simulink model "CognitiveOperatorBackup"  (R2017a)
settings: Solver=VariableStepAuto  StartTime=0.0  StopTime=81  RelTol=1e-3
libraries: simulink x1
settings Model: PauseTimes=1  Creator=Igor Khimchenko  LastModifiedBy=Igor Khimchenko

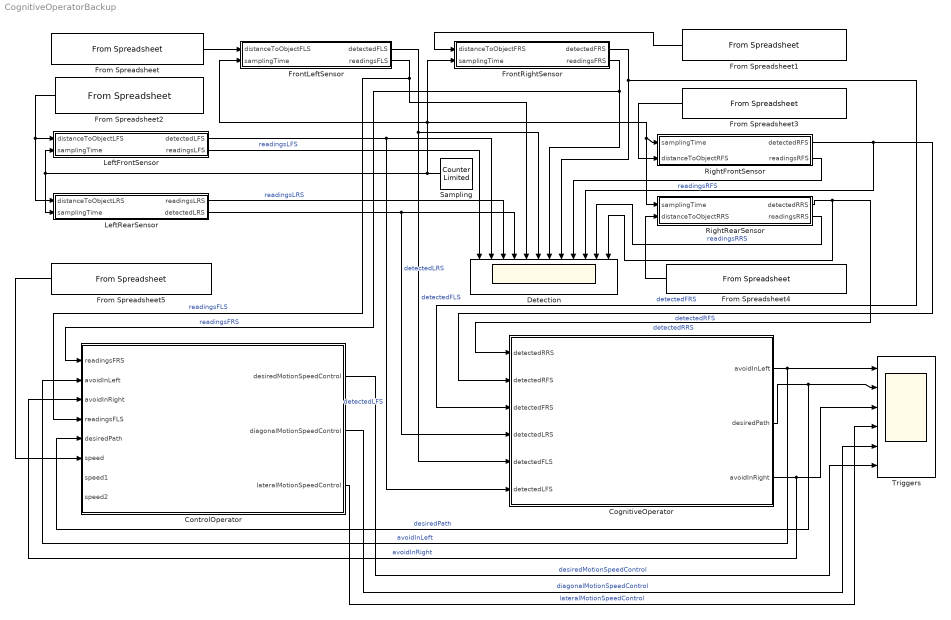
== system CognitiveOperatorBackup ==
  CognitiveOperator : Stateflow chart  TreatAsAtomicUnit=on
  ControlOperator : Stateflow chart  TreatAsAtomicUnit=on
  Detection : Scope  NumInputPorts=12
  From Spreadsheet : FromSpreadsheet  FileName=SensorReadings.xlsx  SheetName=Front left
  From Spreadsheet1 : FromSpreadsheet  FileName=SensorReadings.xlsx  SheetName=Front right
  From Spreadsheet2 : FromSpreadsheet  FileName=SensorReadings.xlsx  SheetName=Left
  From Spreadsheet3 : FromSpreadsheet  FileName=SensorReadings.xlsx  SheetName=Right front
  From Spreadsheet4 : FromSpreadsheet  FileName=SensorReadings.xlsx  SheetName=Right rear
  From Spreadsheet5 : FromSpreadsheet  FileName=SensorReadings.xlsx  SheetName=Speed
  FrontLeftSensor : Stateflow chart  TreatAsAtomicUnit=on
  FrontRightSensor : Stateflow chart  TreatAsAtomicUnit=on
  LeftFrontSensor : Stateflow chart  TreatAsAtomicUnit=on
  LeftRearSensor : Stateflow chart  TreatAsAtomicUnit=on
  RightFrontSensor : Stateflow chart  TreatAsAtomicUnit=on
  RightRearSensor : Stateflow chart  TreatAsAtomicUnit=on
  Sampling : simulink/Sources/Counter Limited  uplimit=50  tsamp=0.001
  Triggers : Scope  NumInputPorts=6
  wires:
  From Spreadsheet2/1 -> LeftRearSensor/1(distanceToObjectLRS), LeftFrontSensor/1(distanceToObjectLFS)
  Sampling/1 -> LeftRearSensor/2(samplingTime), LeftFrontSensor/2(samplingTime), FrontRightSensor/2(samplingTime), RightRearSensor/1(samplingTime), RightFrontSensor/1(samplingTime), FrontLeftSensor/2(samplingTime)
  LeftFrontSensor/2(readingsLFS) -> Detection/1  "readingsLFS"
  LeftFrontSensor/1(detectedLFS) -> CognitiveOperator/6(detectedLFS), Detection/2  "detectedLFS"
  LeftRearSensor/1(readingsLRS) -> Detection/3  "readingsLRS"
  LeftRearSensor/2(detectedLRS) -> CognitiveOperator/4(detectedLRS), Detection/4  "detectedLRS"
  FrontLeftSensor/2(readingsFLS) -> ControlOperator/4(readingsFLS), Detection/5  "readingsFLS"
  FrontLeftSensor/1(detectedFLS) -> CognitiveOperator/5(detectedFLS), Detection/6  "detectedFLS"
  FrontRightSensor/2(readingsFRS) -> ControlOperator/1(readingsFRS), Detection/7  "readingsFRS"
  FrontRightSensor/1(detectedFRS) -> CognitiveOperator/3(detectedFRS), Detection/8  "detectedFRS"
  RightFrontSensor/2(readingsRFS) -> Detection/9  "readingsRFS"
  RightFrontSensor/1(detectedRFS) -> Detection/10, CognitiveOperator/2(detectedRFS)  "detectedRFS"
  RightRearSensor/2(readingsRRS) -> Detection/11  "readingsRRS"
  RightRearSensor/1(detectedRRS) -> CognitiveOperator/1(detectedRRS), Detection/12  "detectedRRS"
  CognitiveOperator/1(avoidInLeft) -> ControlOperator/2(avoidInLeft), Triggers/1  "avoidInLeft"
  CognitiveOperator/2(desiredPath) -> ControlOperator/5(desiredPath), Triggers/2  "desiredPath"
  CognitiveOperator/3(avoidInRight) -> ControlOperator/3(avoidInRight), Triggers/3  "avoidInRight"
  From Spreadsheet3/1 -> RightFrontSensor/2(distanceToObjectRFS)
  From Spreadsheet4/1 -> RightRearSensor/2(distanceToObjectRRS)
  ControlOperator/1(desiredMotionSpeedControl) -> Triggers/6  "desiredMotionSpeedControl"
  ControlOperator/3(lateralMotionSpeedControl) -> Triggers/4  "lateralMotionSpeedControl"
  From Spreadsheet5/1 -> ControlOperator/6(speed)
  From Spreadsheet/1 -> FrontLeftSensor/1(distanceToObjectFLS)
  From Spreadsheet1/1 -> FrontRightSensor/1(distanceToObjectFRS)
  ControlOperator/2(diagonalMotionSpeedControl) -> Triggers/5  "diagonalMotionSpeedControl"

== stateflow chart CognitiveOperatorBackup/LeftFrontSensor ==
  state LFSEnvironmentSampling
    entry: detectedLFS = 0
    readingsLFS = distanceToObjectLFS
  state LFSObstacleDetected
    entry: detectedLFS = 1
    readingsLFS = distanceToObjectLFS
  (default) -> LFSEnvironmentSampling
  LFSEnvironmentSampling -> LFSEnvironmentSampling [order 2] : [samplingTime == 50]
  LFSEnvironmentSampling -> LFSObstacleDetected [order 1] : [distanceToObjectLFS <= 1]
  LFSObstacleDetected -> LFSEnvironmentSampling [order 1] : [not(distanceToObjectLFS <= 1)]
  LFSObstacleDetected -> LFSObstacleDetected [order 2] : [samplingTime == 50]
  data: distanceToObjectLFS input; samplingTime input; detectedLFS output; readingsLFS output

== stateflow chart CognitiveOperatorBackup/LeftRearSensor ==
  state LRSEnvironmentSampling
    entry: detectedLRS = 0
    readingsLRS = distanceToObjectLRS
  state LRSObstacleDetected
    entry: detectedLRS = 1
    readingsLRS = distanceToObjectLRS
  (default) -> LRSEnvironmentSampling
  LRSEnvironmentSampling -> LRSEnvironmentSampling [order 2] : [samplingTime == 50]
  LRSEnvironmentSampling -> LRSObstacleDetected [order 1] : [distanceToObjectLRS <= 1]
  LRSObstacleDetected -> LRSEnvironmentSampling [order 1] : [not(distanceToObjectLRS <= 1)]
  LRSObstacleDetected -> LRSObstacleDetected [order 2] : [samplingTime == 50]
  data: distanceToObjectLRS input; samplingTime input; readingsLRS output; detectedLRS output

== stateflow chart CognitiveOperatorBackup/CognitiveOperator ==
  state DesiredPathTrigger
    entry: avoidInLeft = 0
    avoidInRight = 0
    desiredPath = 1
  state AvoidInLeftTrigger
    entry: avoidInLeft = 1
    avoidInRight = 0
    desiredPath = 0
  state AvoidInRightTrigger
    entry: avoidInLeft = 0
    avoidInRight = 1
    desiredPath = 0
  (default) -> DesiredPathTrigger
  DesiredPathTrigger -> AvoidInLeftTrigger [order 2] : [not(detectedLRS && detectedLFS) && (detectedFLS && detectedFRS) && (detectedRFS && detectedRRS)]
  DesiredPathTrigger -> AvoidInRightTrigger [order 1] : [not(detectedRRS && detectedRFS) && (detectedFLS && detectedFRS) && (detectedLFS && detectedLRS)]
  AvoidInLeftTrigger -> DesiredPathTrigger : [not(detectedFLS) && not(detectedFRS)]
  AvoidInRightTrigger -> DesiredPathTrigger : [not(detectedFLS) && not(detectedFRS)]
  data: detectedRRS input; detectedRFS input; detectedFRS input; detectedLRS input; detectedFLS input; detectedLFS input; avoidInLeft output; desiredPath output; avoidInRight output

== stateflow chart CognitiveOperatorBackup/FrontLeftSensor ==
  state FLSEnvironmentSampling
    entry: detectedFLS = 0
    readingsFLS = distanceToObjectFLS
  state FLSObstacleDetected
    entry: detectedFLS = 1
    readingsFLS = distanceToObjectFLS
  (default) -> FLSEnvironmentSampling
  FLSEnvironmentSampling -> FLSEnvironmentSampling [order 2] : [samplingTime == 50]
  FLSEnvironmentSampling -> FLSObstacleDetected [order 1] : [distanceToObjectFLS <= 1]
  FLSObstacleDetected -> FLSEnvironmentSampling [order 1] : [not(distanceToObjectFLS <= 1)]
  FLSObstacleDetected -> FLSObstacleDetected [order 2] : [samplingTime == 50]
  data: distanceToObjectFLS input; samplingTime input; detectedFLS output; readingsFLS output

== stateflow chart CognitiveOperatorBackup/FrontRightSensor ==
  state FRSEnvironmentSampling
    entry: detectedFRS = 0
    readingsFRS = distanceToObjectFRS
  state FRSObstacleDetected
    entry: detectedFRS = 1
    readingsFRS = distanceToObjectFRS
  (default) -> FRSEnvironmentSampling
  FRSEnvironmentSampling -> FRSEnvironmentSampling [order 2] : [samplingTime == 50]
  FRSEnvironmentSampling -> FRSObstacleDetected [order 1] : [distanceToObjectFRS <= 1]
  FRSObstacleDetected -> FRSEnvironmentSampling [order 1] : [not(distanceToObjectFRS <= 1)]
  FRSObstacleDetected -> FRSObstacleDetected [order 2] : [samplingTime == 50]
  data: distanceToObjectFRS input; samplingTime input; detectedFRS output; readingsFRS output

== stateflow chart CognitiveOperatorBackup/RightFrontSensor ==
  state RFSEnvironmentSampling
    entry: detectedRFS = 0
    readingsRFS = distanceToObjectRFS
  state RFSObstacleDetected
    entry: detectedRFS = 1
    readingsRFS = distanceToObjectRFS
  (default) -> RFSEnvironmentSampling
  RFSEnvironmentSampling -> RFSEnvironmentSampling [order 2] : [samplingTime == 50]
  RFSEnvironmentSampling -> RFSObstacleDetected [order 1] : [distanceToObjectRFS <= 1]
  RFSObstacleDetected -> RFSEnvironmentSampling [order 1] : [not(distanceToObjectRFS <= 1)]
  RFSObstacleDetected -> RFSObstacleDetected [order 2] : [samplingTime == 50]
  data: samplingTime input; distanceToObjectRFS input; detectedRFS output; readingsRFS output

== stateflow chart CognitiveOperatorBackup/RightRearSensor ==
  state RRSEnvironmentSampling
    entry: detectedRRS = 0
    readingsRRS = distanceToObjectRRS
  state RRSObstacleDetected
    entry: detectedRRS = 1
    readingsRRS = distanceToObjectRRS
  (default) -> RRSEnvironmentSampling
  RRSEnvironmentSampling -> RRSEnvironmentSampling [order 2] : [samplingTime == 50]
  RRSEnvironmentSampling -> RRSObstacleDetected [order 1] : [distanceToObjectRRS <= 1]
  RRSObstacleDetected -> RRSEnvironmentSampling [order 1] : [not(distanceToObjectRRS <= 1)]
  RRSObstacleDetected -> RRSObstacleDetected [order 2] : [samplingTime == 50]
  data: samplingTime input; distanceToObjectRRS input; detectedRRS output; readingsRRS output

== stateflow chart CognitiveOperatorBackup/ControlOperator ==
  state LateralMotionSpeedControl
    entry: lateralMotionSpeedControl = 1
    desiredMotionSpeedControl = 0
    diagonalMotionSpeedControl = 0
  state DesiredMotionSpeedControl
    entry: lateralMotionSpeedControl = 0
    desiredMotionSpeedControl = 1
    diagonalMotionSpeedControl = 0
  state DiagonalMotionSpeedControl
    entry: lateralMotionSpeedControl = 0
    desiredMotionSpeedControl = 0
    diagonalMotionSpeedControl = 1
  (default) -> DesiredMotionSpeedControl
  DesiredMotionSpeedControl -> LateralMotionSpeedControl [order 1] : [(avoidInLeft | avoidInRight) & (readingsFLS < 0.3 & readingsFRS < 0.3) & speed == 0]
  DesiredMotionSpeedControl -> DiagonalMotionSpeedControl [order 2] : [(avoidInLeft | avoidInRight) & (readingsFLS < 0.2 | readingsFRS <  0.2 ) & not(readingsFLS <  0.2 & readingsFRS < 0.2) & speed == 0]
  DiagonalMotionSpeedControl -> DesiredMotionSpeedControl : [desiredPath & speed == 0]
  LateralMotionSpeedControl -> DesiredMotionSpeedControl : [desiredPath & speed == 0]
  data: readingsFRS input; avoidInLeft input; avoidInRight input; readingsFLS input; desiredPath input; speed input; desiredMotionSpeedControl output; diagonalMotionSpeedControl output; lateralMotionSpeedControl output; speed1 input; speed2 input
